simulink model "Linearizzazione_fellata_lmi"  (R2025b)
settings: Solver=VariableStepAuto  StartTime=0.0  StopTime=10.0  RelTol=1e-3
undefined symbols (not defined in the file): A, B, C, Comp, K_lmi, nu, nx, x0
settings Model: Creator=Miche  LastModifiedBy=Miche

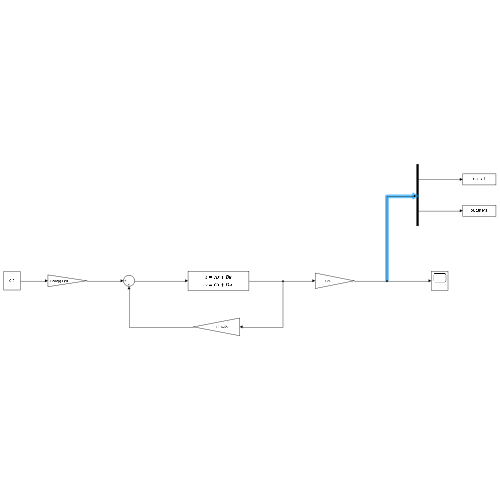
[thumbnail: Simulink's stored preview of the top-level diagram]
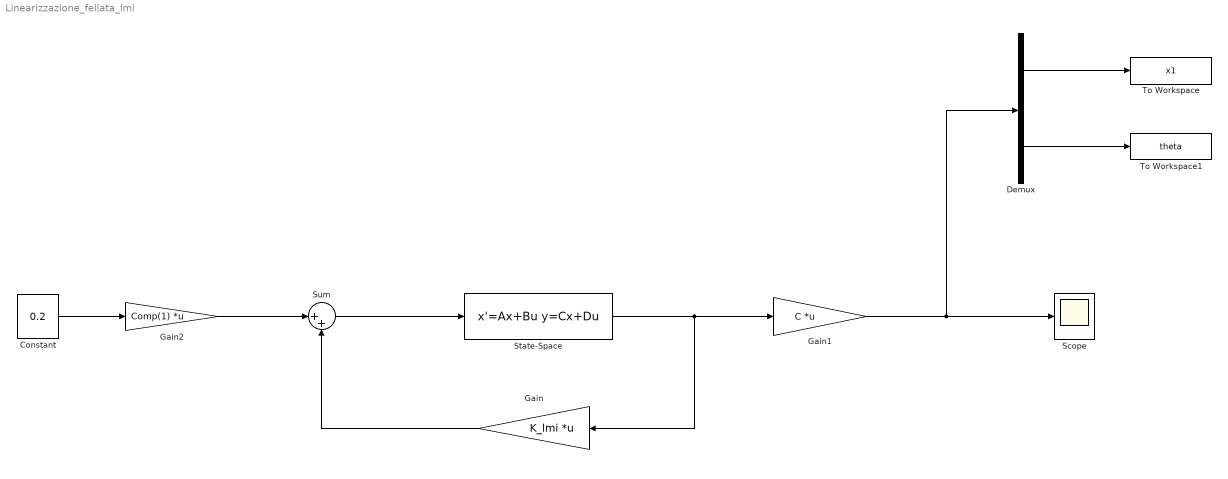
== system Linearizzazione_fellata_lmi ==
  Constant : Constant  Value=0.2
  Demux : Demux  Outputs=2
  Gain : Gain  Gain=K_lmi  Multiplication=Matrix(K*u)
  Gain1 : Gain  Gain=C  Multiplication=Matrix(K*u)
  Gain2 : Gain  Gain=Comp(1)  Multiplication=Matrix(K*u)
  Scope : Scope
      settings: ActiveDisplayYMinimum=-0.13627866165476515  ActiveDisplayYMaximum=0.54080617836899136
  State-Space : StateSpace  A=A  B=B  C=eye(nx)  D=zeros(nx,nu)  InitialCondition=x0
  Sum : Sum  Inputs=|++
  To Workspace : ToWorkspace  VariableName=x1  SaveFormat=Timeseries  SampleTime=-1
  To Workspace1 : ToWorkspace  VariableName=theta  SaveFormat=Timeseries  SampleTime=-1
  wires:
  Sum/1 -> State-Space/1
  Gain/1 -> Sum/2
  State-Space/1 -> Gain/1, Gain1/1
  Gain2/1 -> Sum/1
  Constant/1 -> Gain2/1
  Demux/1 -> To Workspace/1
  Gain1/1 -> Demux/1, Scope/1
  Demux/2 -> To Workspace1/1
